simulink model "MatlabFunctionBlockTestModel"  (R2015a)
settings: Solver=VariableStepDiscrete  StartTime=0.0  StopTime=10.0  RelTol=1e-3
settings Model: Creator=tsprock3  LastModifiedBy=tsprock3
settings SolverCC: MaxConsecutiveZCs=10000

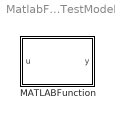
== system MatlabFunctionBlockTestModel ==
  MATLABFunction : MATLAB Function  TreatAsAtomicUnit=on

== matlab function MatlabFunctionBlockTestModel/MATLABFunction ==
  data: u input; y output
function y = fcn(u)
%#codegen

y = u;
